simulink model "pid_motor_real"  (R2015b)
settings: Solver=VariableStepAuto  StartTime=0.0  StopTime=6  RelTol=1e-3
settings Model: Creator=nico  LastModifiedBy=nico

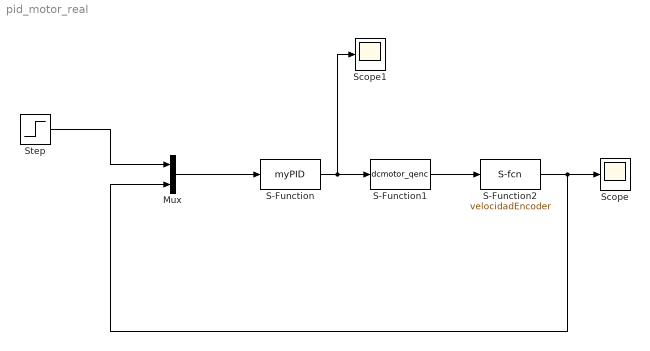
== system pid_motor_real ==
  Mux : Mux  Inputs=2
  S-Function : S-Function  FunctionName=myPID  Parameters=1.2 0.0002 10 10 .0001 0 24  SFunctionDeploymentMode=off  EnableBusSupport=off
  S-Function1 : S-Function  FunctionName=dcmotor_qenc  Parameters=1  SFunctionDeploymentMode=off  EnableBusSupport=off
  S-Function2 : S-Function  FunctionName=velocidadEncoder  Parameters=1 0.0001  SFunctionDeploymentMode=off  EnableBusSupport=off
  Scope : Scope
  Scope1 : Scope
  Step : Step  Time=0.2  After=50  SampleTime=0
  wires:
  Mux/1 -> S-Function/1
  Step/1 -> Mux/1
  S-Function/1 -> Scope1/1, S-Function1/1
  S-Function1/1 -> S-Function2/1
  S-Function2/1 -> Mux/2, Scope/1
